simulink model "PWM_controlPar_Observador"  (R2020b)
settings: Solver=ode15s  StartTime=0.0  StopTime=10.0  FixedStep=0.01  RelTol=1e-3
undefined symbols (not defined in the file or in its folder): X, Y, Z
libraries: fl_lib x8, nesl_utility x6, sm_lib x5, ee_lib x3
settings Model: Creator=petir  LastModifiedBy=petir

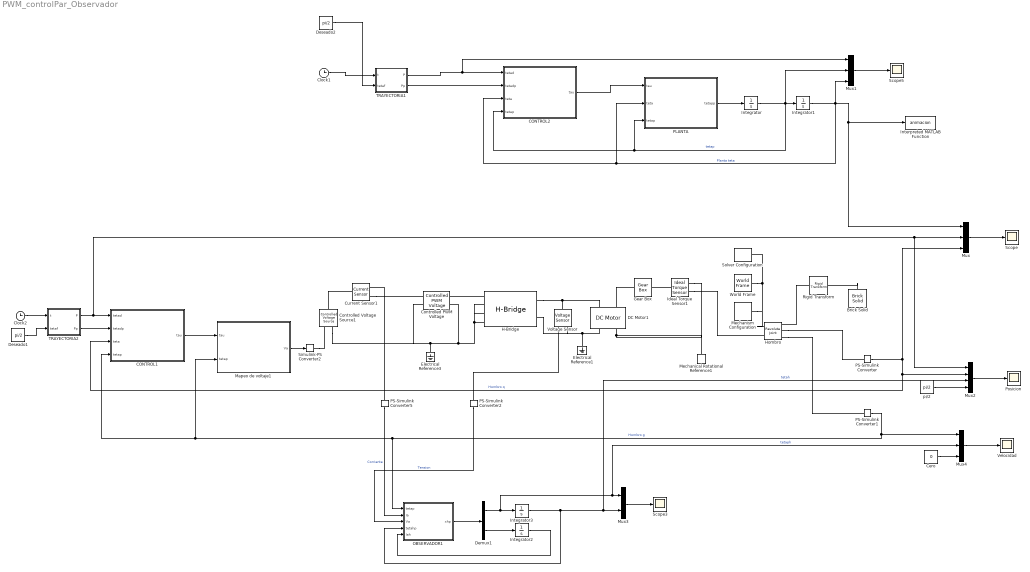
== system PWM_controlPar_Observador ==
  Brick Solid : sm_lib/Body Elements/Brick Solid  GraphicAmbientColor=[0.15 0.15 0.15 1.0]  BasedOnType=Density  BrickDimensions=[0.05 0.5 0.05]  BrickDimensionUnits=m  CenterOfMass=[0 0 0]  CenterOfMassUnits=m  GraphicDiffuseColor=[0.5 0.5 0.5]  Density=1000  DensityUnits=kg/m^3  DoExposeReferenceFrame=on  GraphicEmissiveColor=[0.0 0.0 0.0 1.0]  ExportEntireGeometry=off  SerializedFrames=<Frames/>  MarkerShape=Sphere  MarkerSize=10  GraphicType=FromGeometry  InertiaType=Custom  Mass=0.3  MassUnits=kg  MomentsOfInertia=[1 1 0.002547]  MomentsOfInertiaUnits=kg*m^2  GraphicOpacity=1.0  ProductsOfInertia=[0 0 0]  ProductsOfInertiaUnits=kg*m^2  GraphicShininess=75  GraphicSpecularColor=[0.5 0.5 0.5 1.0]  GraphicVisPropType=SimpleVisualProperties
      settings: SourceProductName=Multibody
  CONTROL1 : MATLAB Function  TreatAsAtomicUnit=on
  CONTROL2 : MATLAB Function  TreatAsAtomicUnit=on
  Cero : Constant  Value=0  VectorParams1D=off
  Clock1 : Clock
  Clock2 : Clock
  Controlled PWM Voltage : ee_lib/Integrated Circuits/Controlled PWM Voltage  F=2000 Hz  TD=0 s  pulse_width_offset=0 s  pulse_min=0 s  Vmin=0 V  Vmax=5 V  Vm=5 V  pwm_or_av=2  event_type=1  sample_time=1e-6 s  u_min=0  u_max=1
  Controlled Voltage Source1 : fl_lib/Electrical/Electrical Sources/Controlled Voltage Source
  Current Sensor1 : fl_lib/Electrical/Electrical Sensors/Current Sensor
  DC Motor1 : ee_lib/Electromechanical/Brushed Motors/DC Motor  field_option=ee.enum.field_option.pm  Rf=100 Ohm  Lf=1 H  Laf=0.15 H  If0=0 A  parameterization=ee.enum.dcparam_option.circuit_param  Ra=8.3 Ohm  La=1.51e-3 H  emf_or_torque=ee.enum.emf_or_torque.ki  Kv=0.072e-3 V/rpm  Ki=0.0879 N*m/A  T_stall=0.24e-3 N*m  w_max=19100 rpm  w_rated=15000 rpm  P_rated=0.08 W  V_rated=1.5 V  J=80.7e-6 kg*m^2  lam_param=ee.enum.lam_param.damping  lam=14.41e-6 N*m/(rad/s)  i_noload=0 A  V_i_noload=1.5 V  speed0=0 rpm  enable_fault_armature=ee.enum.faults.faultEnable.no  rev_faulted=1 / 3  G_faulted_armature=1e-5 S  fault_trigger_armature=ee.enum.faults.faultTrigger.temporal  t_fault_armature=1 s  max_permissible_current_armature=inf A  t_fail_on_current_armature=1 s  enable_fault_field=ee.enum.faults.faultEnable.no  G_faulted_field=1e-5 S  fault_trigger_field=ee.enum.faults.faultTrigger.temporal  t_fault_field=1 s  max_permissible_current_field=inf A  t_fail_on_current_field=1 s  fault_action=ee.enum.faults.faultAction.none  alpha=3.93e-3 1/K  Tmeas=25 degC  thermal_mass=100 J/K  initial_temperature=25 degC
  Demux1 : Demux  Outputs=2
  Deseado1 : Constant  Value=pi/2  VectorParams1D=off
  Deseado2 : Constant  Value=pi/2  VectorParams1D=off
  Electrical Reference1 : fl_lib/Electrical/Electrical Elements/Electrical Reference
  Electrical Reference3 : fl_lib/Electrical/Electrical Elements/Electrical Reference
  Gear Box : fl_lib/Mechanical/Mechanisms/Gear Box  ratio=64  t_in_specify=off  t_in_priority=None  t_in=0 N*m  t_in_nominal_specify=off  t_in_nominal_unit=N*m  t_in_nominal_value=1  t_out_specify=off  t_out_priority=None  t_out=0 N*m  t_out_nominal_specify=off  t_out_nominal_unit=N*m  t_out_nominal_value=1
  H-Bridge : ee_lib/Semiconductors & Converters/Converters/H-Bridge  supply_ports=ee.enum.supply_ports.hidesupply  Venable=2.5 V  Vmax=5 V  Vreverse=2.5 V  Vbrake=2.5 V  Vm=10 V  pwm_or_av=ee.enum.pwm_or_av.averaged  regenerative_braking_mode=ee.enum.converters.regenerative_braking_mode.depends_on_rev  discontinuous=ee.enum.current_profile.continuous  freewheeling_mode=ee.enum.converters.freewheeling_mode.one_switch_one_diode  Ron=0.1 Ohm  Don=0.05 Ohm  Goff=1e-6 S  Rload=10 Ohm  Lload=1e-5 H  F=10 kHz  thermal_mass=100 J/K  initial_temperature=298.15 K  Ron2=0.1 Ohm  Don2=0.05 Ohm  Tmeas=298.15 K  Tmeas2=398.15 K
  Hombro : sm_lib/Joints/Revolute Joint  JointMode=Normal  SenseConstraintForce=off  SenseConstraintForceX=off  SenseConstraintForceY=off  SenseConstraintForceZ=off  SenseConstraintTorque=off  SenseConstraintTorqueX=off  SenseConstraintTorqueY=off  SenseConstraintTorqueZ=off  SenseTotalForce=off  SenseTotalForceX=off  SenseTotalForceY=off  SenseTotalForceZ=off  SenseTotalTorque=off  SenseTotalTorqueX=off  SenseTotalTorqueY=off  SenseTotalTorqueZ=off  CompositeWrenchDir=FollowerOnBase  CompositeWrenchFrame=BaseFrame  EquilibriumPosition=0  EquilibriumPositionUnits=deg  SpringStiffness=0  SpringStiffnessUnits=N*m/deg  DampingCoefficient=0.0017  DampingCoefficientUnits=N*m/(rad/s)  TorqueActuationMode=InputTorque  MotionActuationMode=ComputedMotion  SensePosition=on  SenseVelocity=on  SenseAcceleration=off  SenseTorqueForce=off  SenseLowerLimitTorqueForce=off  SenseUpperLimitTorqueForce=off  LowerLimitSpecify=off  LowerLimitBound=-90  LowerLimitBoundUnits=deg  LowerLimitStiffness=1e4  LowerLimitStiffnessUnits=N*m/deg  LowerLimitDamping=10  LowerLimitDampingUnits=N*m/(deg/s)  LowerLimitTransitionRegionWidth=0.1  LowerLimitTransitionRegionWidthUnits=deg  UpperLimitSpecify=off  UpperLimitBound=90  UpperLimitBoundUnits=deg  UpperLimitStiffness=1e4  UpperLimitStiffnessUnits=N*m/deg  UpperLimitDamping=10  UpperLimitDampingUnits=N*m/(deg/s)  UpperLimitTransitionRegionWidth=0.1  UpperLimitTransitionRegionWidthUnits=deg  PositionTargetSpecify=off  PositionTargetPriority=High  PositionTargetValue=0  PositionTargetValueUnits=deg  VelocityTargetSpecify=off  VelocityTargetPriority=High  VelocityTargetValue=0  VelocityTargetValueUnits=deg/s
  Ideal Torque Sensor1 : fl_lib/Mechanical/Mechanical Sensors/Ideal Torque Sensor
  Integrator{,1..3} (4 alike) : Integrator
  Interpreted MATLAB Function : MATLABFcn  MATLABFcn=animacion
  Mapeo de voltaje1 : MATLAB Function  TreatAsAtomicUnit=on
  Mechanical Rotational Reference1 : fl_lib/Mechanical/Rotational Elements/Mechanical Rotational Reference
  Mechanism Configuration : sm_lib/Utilities/Mechanism Configuration  UniformGravity=Constant  GravityVector=[0 -9.80665 0]  GravityVectorUnits=m/s^2  GravityUnits=m/s^2  LinearizationDelta=0.001  JointModeTransitionNonlinearIterations=2
      settings: SourceProductName=Multibody
  Mux : Mux  Inputs=3
  Mux1 : Mux  Inputs=3
  Mux2 : Mux
  Mux3 : Mux  Inputs=2
  Mux4 : Mux  Inputs=3
  OBSERVADOR1 : MATLAB Function  TreatAsAtomicUnit=on
  PLANTA : MATLAB Function  TreatAsAtomicUnit=on
  PS-Simulink Converter{,1..2,5} (4 alike) : nesl_utility/PS-Simulink Converter  PhysicalDomain=network_engine_domain  SubClassName=ps_output  LeftPortType=input  RightPortType=output  PseudoPeriodic=off  Frequencies=[]  Unit=inherit  AffineConversion=off
      PS-Simulink Converter settings: SourceProductName=Utilities
      PS-Simulink Converter1 settings: SourceProductName=Utilities
  Posicion : Scope
  Rigid Transform : sm_lib/Frames and Transforms/Rigid Transform  TranslationMethod=Cartesian  TranslationStandardOffset=0  TranslationLengthUnit=m  TranslationStandardAxis=+Z  TranslationCartesianOffset=[0 -0.25 0]  TranslationROffset=0  TranslationROffsetUnits=m  TranslationZOffset=0  TranslationZOffsetUnits=m  TranslationThetaOffset=0  TranslationThetaOffsetUnits=deg  RotationMethod=None  RotationAngleUnits=deg  RotationStandardAxis=+Z  RotationAngle=0.0  RotationArbitraryAxis=[0 0 1]  FollAlignAxisA=+X  BaseAlignAxisA=+Y  FollAlignAxisB=+Y  BaseAlignAxisB=+Z  RotationSequenceAxes=FollowerAxes  RotationSequence=XYX  RotationSequenceAngles=[0 0 0]  RotationSequenceAnglesUnits=deg  RotationMatrix=[1 0 0; 0 1 0; 0 0 1]
      settings: SourceProductName=Multibody
  Scope : Scope
  Scope3 : Scope
  Scope5 : Scope
  Simulink-PS Converter2 : nesl_utility/Simulink-PS Converter  PhysicalDomain=network_engine_domain  SubClassName=ps_input  LeftPortType=input  RightPortType=output  PseudoPeriodic=off  Frequencies=[]  NoiseDistribution=none  NoiseParameters=[]  Unit=1  AffineConversion=off  FilteringAndDerivatives=provide  SimscapeFilterOrder=1  InputFilterTimeConstant=0.001  UdotUserProvided=0
      settings: SourceProductName=Utilities
  Solver Configuration : nesl_utility/Solver Configuration  PhysicalDomain=network_engine_domain  SubClassName=solver  LeftPortType=input  RightPortType=generic  Tones=[]  Harmonics=[]  SimulateNoise=off  Profile=off  UseLocalSampling=off  EnableSwitchedLinearOptims=on  FrequencyDomain=off  UseCCode=off  RelTol=0.001  AbsTol=1e-06  MinStep=1e-09  ToWorkspace=off  RevertToSquareIcSolve=off  NumHomotopyIterations=100  PhasorMode=off  PhasorModeNumHarmonics=1  DoDC=off  ResidualTolerance=1e-09  UseLocalSolver=off  LocalSolverChoice=NE_BACKWARD_EULER_ADVANCER  LocalSolverSampleTime=0.001  DoFixedCost=off  MaxNonlinIter=3  MaxModeIter=2  ComputeImpulses=off  ImpulseIterations=2  LinearAlgebra=Sparse  EquationFormulation=NE_TIME_EF  DelaysMemoryBudget=1024  AutomaticFiltering=on  FilteringTimeConstant=0.001  PartitionStorageMethod=AS_NEEDED  PartitionMemoryBudget=1024  PartitionMethod=FAST
      settings: SourceProductName=Utilities
  TRAYECTORIA1 : MATLAB Function  TreatAsAtomicUnit=on
  TRAYECTORIA2 : MATLAB Function  TreatAsAtomicUnit=on
  Velocidad : Scope
  Voltage Sensor : fl_lib/Electrical/Electrical Sensors/Voltage Sensor
  World Frame : sm_lib/Frames and Transforms/World Frame
      settings: SourceProductName=Multibody
  pi/2 : Constant  Value=pi/2  VectorParams1D=off
  wires:
  PLANTA/1(tetapp) -> Integrator/1
  Integrator/1 -> Integrator1/1, Mux1/2, CONTROL2/4(tetap), PLANTA/3(tetap)  "tetap"
  Integrator1/1 -> CONTROL2/3(teta), PLANTA/2(teta), Mux1/3, Mux/1, Interpreted MATLAB Function/1  "Planta teta"
  Mux/1 -> Scope/1
  PS-Simulink Converter1/1 -> CONTROL1/4(tetap), Mapeo de voltaje1/2(tetap), OBSERVADOR1/1(tetap), Mux4/1  "Hombro g"
  CONTROL1/1(tau) -> Mapeo de voltaje1/1(tau)
  PS-Simulink Converter/1 -> Mux/3, CONTROL1/3(teta), Mux2/2  "Hombro q"
  Deseado2/1 -> TRAYECTORIA1/2(tetaf)
  TRAYECTORIA1/1(P) -> Mux1/1, CONTROL2/1(tetad)
  Clock1/1 -> TRAYECTORIA1/1(t)
  CONTROL2/1(tau) -> PLANTA/1(tau)
  TRAYECTORIA1/2(Pp) -> CONTROL2/2(tetadp)
  Mux1/1 -> Scope5/1
  Deseado1/1 -> TRAYECTORIA2/2(tetaf)
  TRAYECTORIA2/2(Pp) -> CONTROL1/2(tetadp)
  Clock2/1 -> TRAYECTORIA2/1(t)
  TRAYECTORIA2/1(P) -> CONTROL1/1(tetad), Mux2/1, Mux/2
  Mapeo de voltaje1/1(Va) -> Simulink-PS Converter2/1
  Demux1/1 -> Mux4/2, Mux3/1, Integrator3/1  "tetaph"
  Demux1/2 -> Integrator2/1
  PS-Simulink Converter5/1 -> OBSERVADOR1/2(Ia)  "Corriente"
  OBSERVADOR1/1(xhp) -> Demux1/1
  Integrator3/1 -> Mux2/3, Mux3/2, OBSERVADOR1/4(tetahp)  "tetah"
  Integrator2/1 -> OBSERVADOR1/5(Iah)
  Mux3/1 -> Scope3/1
  Mux4/1 -> Velocidad/1
  PS-Simulink Converter2/1 -> OBSERVADOR1/3(Va)  "Tension"
  Mux2/1 -> Posicion/1
  pi/2/1 -> Mux2/4
  Cero/1 -> Mux4/3
  connections:
  World Frame/RConn1 -- Solver Configuration/RConn1 -- Hombro/LConn1 -- Mechanism Configuration/RConn1
  Rigid Transform/LConn1 -- Hombro/RConn1
  Hombro/RConn3 -- PS-Simulink Converter1/LConn1
  Brick Solid/RConn1 -- Rigid Transform/RConn1
  Hombro/RConn2 -- PS-Simulink Converter/LConn1
  Electrical Reference1/LConn1 -- H-Bridge/RConn2 -- Voltage Sensor/RConn2 -- DC Motor1/RConn1
  DC Motor1/RConn2 -- Ideal Torque Sensor1/RConn1 -- Mechanical Rotational Reference1/LConn1
  Ideal Torque Sensor1/LConn1 -- Gear Box/RConn1
  Gear Box/LConn1 -- DC Motor1/LConn2
  Simulink-PS Converter2/RConn1 -- Controlled Voltage Source1/RConn1
  Ideal Torque Sensor1/RConn2 -- Hombro/LConn2
  H-Bridge/LConn1 -- Controlled PWM Voltage/RConn1
  H-Bridge/LConn4 -- Controlled Voltage Source1/RConn2 -- Controlled PWM Voltage/LConn2 -- Electrical Reference3/LConn1 -- Controlled PWM Voltage/RConn2 -- H-Bridge/LConn2 -- H-Bridge/LConn3
  Current Sensor1/RConn2 -- Controlled PWM Voltage/LConn1
  PS-Simulink Converter5/LConn1 -- Current Sensor1/RConn1
  H-Bridge/RConn1 -- Voltage Sensor/LConn1 -- DC Motor1/LConn1
  Current Sensor1/LConn1 -- Controlled Voltage Source1/LConn1
  PS-Simulink Converter2/LConn1 -- Voltage Sensor/RConn1

== matlab function PWM_controlPar_Observador/CONTROL2 ==
  data: tetad input; tetadp input; tau output; teta input; tetap input
function tau  = fcn(tetad, tetadp, teta, tetap)
% Parametros
m = 0.3;
lc = 0.25;
I = 0.002547;
Bf = 0.0017;
g = 9.81;

% tetad =  pi / 2;
Kd = 2;
Kp = 15;

Vaux = Kp * (tetad - teta) - Kd * (tetap);
tau = 1 / (m * lc^2 + I) * Vaux + Bf * (tetap) - m * g * lc * sin(teta);

== matlab function PWM_controlPar_Observador/PLANTA ==
  data: tau input; tetapp output; teta input; tetap input
function tetapp = fcn(tau, teta, tetap)
% Parametros
m = 0.3;
lc = 0.25;
I = 0.002547;
Bf = 0.0017;
g = 9.81;

tetapp = 1 / (m * lc^2 + I) * (tau - Bf * tetap - m * g * lc * sin(teta));

== matlab function PWM_controlPar_Observador/CONTROL1 ==
  data: tetad input; tetadp input; tau output; teta input; tetap input
function tau  = fcn(tetad, tetadp, teta, tetap)
% Parametros
m = 0.3;
lc = 0.25;
I = 0.002547;
Bf = 0.0017;
g = 9.81;

gearRatio = 64*1.6;
% tetad =  pi / 2;
Kd = 2;
Kp = 15;

Vaux = Kp * (tetad - teta) - Kd * (tetap);
tau = 1 / (m * lc^2 + I) * Vaux + Bf * tetap - m * g * lc * sin(teta/gearRatio);

== matlab function PWM_controlPar_Observador/OBSERVADOR1 ==
  data: tetap input; Ia input; Va input; xhp output; tetahp input; Iah input
function xhp = fcn(tetap, Ia, Va, tetahp, Iah)
% Parámetros
Ra = 8.3;
La = 1.51e-3;
Ke = 0.0879;
Ki = 0.0879;
J = 80.7e-6;
B = 14.41e-6;
TL = 0.1;

% Planta
% tetapp = Ki / (J * Ra) * Va - Ki * Ke / (J * Ra) * tetap - B / J * tetap - 1 / J * TL;

A = [-B / J, Ki / J; -Ke/La, -Ra / La];
B_mat = [0; 1 / La];
C = [0, 1];

x = [tetap; Ia];
xh = [tetahp; Iah];

y = C * x;
yh = C * xh;

% K = [-1087.5267; -5476.89*];
% K = [19.8214*50; 96.8214*1000];
K = [19.8214*50; 96.8214*1250];
% K = [1; 1]
% xph = Axh + Bu + k(y-yh)
xhp = A * xh + B_mat * Va + K * (y - yh);

== matlab function PWM_controlPar_Observador/TRAYECTORIA2 ==
  data: t input; P output; Pp output; tetaf input
function [P, Pp] = fcn(t, tetaf)
% Parametros
teta0 = 0;
tetap0 = 0;
tetapf = 0;
% Tiempo de simulación
tf = 10;

P = teta0 + tetap0 * t + (3/tf^2) * (tetaf - teta0) * t^2 - (2/tf^3) * (tetaf - teta0) * t^3;
Pp = teta0 + (6/tf^2) * (tetaf - teta0) * t - (6 / tf^3) * (tetaf - teta0) * t^2;

== matlab function PWM_controlPar_Observador/TRAYECTORIA1 ==
  data: t input; P output; Pp output; tetaf input
function [P, Pp] = fcn(t, tetaf)
% Parametros
teta0 = 0;
tetap0 = 0;
tetapf = 0;
% Tiempo de simulación
tf = 10;

P = teta0 + tetap0 * t + (3/tf^2) * (tetaf - teta0) * t^2 - (2/tf^3) * (tetaf - teta0) * t^3;
Pp = teta0 + (6/tf^2) * (tetaf - teta0) * t - (6 / tf^3) * (tetaf - teta0) * t^2;

== matlab function PWM_controlPar_Observador/Mapeo de voltaje1 ==
  data: Va output; tau input; tetap input
function Va = fcn(tau, tetap)
% Parametros
Ra = 8.3;
Ki = 0.0879;
Ke = 0.0879;

Va = Ra / Ki * tau + Ke * tetap;
